simulink model "CMOS_Kernel_Memory_Sync"  (R2023b)
settings: Solver=VariableStepAuto  StartTime=0.0  StopTime=30000000  RelTol=1e-3
values from neighbouring files (symbols this model uses):
  AmountOfPixelsPerScanline = 400    [Kernel_Setup_Script.m]
  AmountOfRamBlocksScanlines = 5    [Kernel_Setup_Script.m]
  AmountOfRamBlocksScanlinesOffset = AmountOfRamBlocksScanlines - 1    (= 4)    [Kernel_Setup_Script.m]
  AmountOfScanlinePixels = 73700    [Kernel_Setup_Script.m]
  AmountOfScanlinePixelsOffset = AmountOfScanlinePixels - 1    (= 73699)    [Kernel_Setup_Script.m]
  AmountOfScanlines = 1100    [Kernel_Setup_Script.m]
  AmountOfScanlinesOffset = AmountOfScanlines - 1    (= 1099)    [Kernel_Setup_Script.m]
  AOPPK_Off = AmountOfPixelsPerScanline - 1    (= 399)    [Kernel_Setup_Script.m]
  AOPPS_Off = AmountOfPixelsPerScanline - 1    (= 399)    [Kernel_Setup_Script.m]
  FramePackOff_0 = FramePackOff_0 - ScanlineFifoCheck    [Kernel_Setup_Script.m]
  FramePackOff_1 = FramePackOff_1 - ScanlineFifoCheck    [Kernel_Setup_Script.m]
  FramePackOff_2 = FramePackOff_2 - ScanlineFifoCheck    [Kernel_Setup_Script.m]
  FramePackOff_3 = FramePackOff_3 - ScanlineFifoCheck    [Kernel_Setup_Script.m]
  FramePackOff_4 = FramePackOff_4 - ScanlineFifoCheck    [Kernel_Setup_Script.m]
  FramePackOff_5 = FramePackOff_5 - ScanlineFifoCheck    [Kernel_Setup_Script.m]
  KernelPackOff_0 = KernelPackOff_0 - KernelBitsPerRow    [Kernel_Setup_Script.m]
  KernelPackOff_1 = KernelPackOff_1 - KernelBitsPerRow    [Kernel_Setup_Script.m]
  KernelPackOff_2 = KernelPackOff_2 - KernelBitsPerRow    [Kernel_Setup_Script.m]
  KernelPackOff_3 = KernelPackOff_3 - KernelBitsPerRow    [Kernel_Setup_Script.m]
  Slice59DownTo48Top = (MsbOffset - (ScanlinePixelBitSizeController*1))    (= 59)    [Kernel_Setup_Script.m]
  Slice71DownTo60Top = (MsbOffset - (ScanlinePixelBitSizeController*0))    (= 71)    [Kernel_Setup_Script.m]
  TotalSectionsForFrames = AmountOfScanlines/AmountOfRamBlocksScanlines    (= 220)    [Kernel_Setup_Script.m]
  UltraRamRows = AmountOfPixelsPerScanline/ScanlineFifoCheck    [Kernel_Setup_Script.m]
  UltraRamRowsCeil = ceil(AmountOfPixelsPerScanline/ScanlineFifoCheck)    [Kernel_Setup_Script.m]
  UltraRamRowsKernel = AmountOfPixelsPerScanline/KernelBitsPerRow    (= 100)    [Kernel_Setup_Script.m]
  UltraRamRowsKernelCeil = ceil(AmountOfPixelsPerScanline/KernelBitsPerRow)    [Kernel_Setup_Script.m]
  UltraRamRowsMemorySectionOffset = UltraRamRowsCeil*AmountOfRamBlocksScanlines    [Kernel_Setup_Script.m]
  UltraRamRowsOffset = UltraRamRowsCeil - 1    [Kernel_Setup_Script.m]
undefined symbols (not defined in the file or in its folder): c, Down, sfvc784, Up, xck26
libraries: hdlBasic x4512, vmcUtilities x1
(part 38 of 39)

== system CMOS_Kernel_Memory_Sync/Memory Handler/Data Slicer/Kernel RAM Slicer/72 Bit Kernel Unpacker RAM 1/Unpack Kernel 72 Bit FIFO 0 ==
  72 Bit Input : Inport
  Slice 17 Down To 0 : hdlBasic/Slice  nbits=KernelWeightBitSizeController  boolean_output=off  mode=Upper Bit Location + Width  bit1=KernelSlice17DownTo0Top  base1=LSB of Input  bit0=0  base0=Binary Point of Input  XmcBlockStatus=1  maskContainerNames=group1  block_type=slice  block_config=sysgen:Slice_config
  Slice 35 Down To 18 : hdlBasic/Slice  nbits=KernelWeightBitSizeController  boolean_output=off  mode=Upper Bit Location + Width  bit1=KernelSlice35DownTo18Top  base1=LSB of Input  bit0=18  base0=Binary Point of Input  XmcBlockStatus=1  maskContainerNames=group1  block_type=slice  block_config=sysgen:Slice_config
  Slice 53 Down To 36 : hdlBasic/Slice  nbits=KernelWeightBitSizeController  boolean_output=off  mode=Upper Bit Location + Width  bit1=KernelSlice53DownTo36Top  base1=LSB of Input  bit0=36  base0=Binary Point of Input  XmcBlockStatus=1  maskContainerNames=group1  block_type=slice  block_config=sysgen:Slice_config
  Slice 71 Down To 54 : hdlBasic/Slice  nbits=KernelWeightBitSizeController  boolean_output=off  mode=Upper Bit Location + Width  bit1=KernelSlice71DownTo54Top  base1=LSB of Input  bit0=54  base0=Binary Point of Input  XmcBlockStatus=1  maskContainerNames=group1  block_type=slice  block_config=sysgen:Slice_config
  71 Downto 54 : Outport
  53 Downto 36 : Outport  Port=2
  35 Downto 18 : Outport  Port=3
  17 Downto 0 : Outport  Port=4
  wires:
  72 Bit Input/1 -> Slice 17 Down To 0/1, Slice 35 Down To 18/1, Slice 53 Down To 36/1, Slice 71 Down To 54/1
  Slice 35 Down To 18/1 -> 35 Downto 18/1
  Slice 53 Down To 36/1 -> 53 Downto 36/1
  Slice 17 Down To 0/1 -> 17 Downto 0/1
  Slice 71 Down To 54/1 -> 71 Downto 54/1

== system CMOS_Kernel_Memory_Sync/Memory Handler/Data Slicer/Kernel RAM Slicer/72 Bit Kernel Unpacker RAM 1/Unpack Kernel 72 Bit FIFO 1 ==
  72 Bit Input : Inport
  Slice 17 Down To 0 : hdlBasic/Slice  nbits=KernelWeightBitSizeController  boolean_output=off  mode=Upper Bit Location + Width  bit1=KernelSlice17DownTo0Top  base1=LSB of Input  bit0=0  base0=Binary Point of Input  XmcBlockStatus=1  maskContainerNames=group1  block_type=slice  block_config=sysgen:Slice_config
  Slice 35 Down To 18 : hdlBasic/Slice  nbits=KernelWeightBitSizeController  boolean_output=off  mode=Upper Bit Location + Width  bit1=KernelSlice35DownTo18Top  base1=LSB of Input  bit0=18  base0=Binary Point of Input  XmcBlockStatus=1  maskContainerNames=group1  block_type=slice  block_config=sysgen:Slice_config
  Slice 53 Down To 36 : hdlBasic/Slice  nbits=KernelWeightBitSizeController  boolean_output=off  mode=Upper Bit Location + Width  bit1=KernelSlice53DownTo36Top  base1=LSB of Input  bit0=36  base0=Binary Point of Input  XmcBlockStatus=1  maskContainerNames=group1  block_type=slice  block_config=sysgen:Slice_config
  Slice 71 Down To 54 : hdlBasic/Slice  nbits=KernelWeightBitSizeController  boolean_output=off  mode=Upper Bit Location + Width  bit1=KernelSlice71DownTo54Top  base1=LSB of Input  bit0=54  base0=Binary Point of Input  XmcBlockStatus=1  maskContainerNames=group1  block_type=slice  block_config=sysgen:Slice_config
  71 Downto 54 : Outport
  53 Downto 36 : Outport  Port=2
  35 Downto 18 : Outport  Port=3
  17 Downto 0 : Outport  Port=4
  wires:
  72 Bit Input/1 -> Slice 17 Down To 0/1, Slice 35 Down To 18/1, Slice 53 Down To 36/1, Slice 71 Down To 54/1
  Slice 35 Down To 18/1 -> 35 Downto 18/1
  Slice 53 Down To 36/1 -> 53 Downto 36/1
  Slice 17 Down To 0/1 -> 17 Downto 0/1
  Slice 71 Down To 54/1 -> 71 Downto 54/1

== system CMOS_Kernel_Memory_Sync/Memory Handler/Data Slicer/Kernel RAM Slicer/72 Bit Kernel Unpacker RAM 1/Unpack Kernel 72 Bit FIFO 2 ==
  72 Bit Input : Inport
  Slice 17 Down To 0 : hdlBasic/Slice  nbits=KernelWeightBitSizeController  boolean_output=off  mode=Upper Bit Location + Width  bit1=KernelSlice17DownTo0Top  base1=LSB of Input  bit0=0  base0=Binary Point of Input  XmcBlockStatus=1  maskContainerNames=group1  block_type=slice  block_config=sysgen:Slice_config
  Slice 35 Down To 18 : hdlBasic/Slice  nbits=KernelWeightBitSizeController  boolean_output=off  mode=Upper Bit Location + Width  bit1=KernelSlice35DownTo18Top  base1=LSB of Input  bit0=18  base0=Binary Point of Input  XmcBlockStatus=1  maskContainerNames=group1  block_type=slice  block_config=sysgen:Slice_config
  Slice 53 Down To 36 : hdlBasic/Slice  nbits=KernelWeightBitSizeController  boolean_output=off  mode=Upper Bit Location + Width  bit1=KernelSlice53DownTo36Top  base1=LSB of Input  bit0=36  base0=Binary Point of Input  XmcBlockStatus=1  maskContainerNames=group1  block_type=slice  block_config=sysgen:Slice_config
  Slice 71 Down To 54 : hdlBasic/Slice  nbits=KernelWeightBitSizeController  boolean_output=off  mode=Upper Bit Location + Width  bit1=KernelSlice71DownTo54Top  base1=LSB of Input  bit0=54  base0=Binary Point of Input  XmcBlockStatus=1  maskContainerNames=group1  block_type=slice  block_config=sysgen:Slice_config
  71 Downto 54 : Outport
  53 Downto 36 : Outport  Port=2
  35 Downto 18 : Outport  Port=3
  17 Downto 0 : Outport  Port=4
  wires:
  72 Bit Input/1 -> Slice 17 Down To 0/1, Slice 35 Down To 18/1, Slice 53 Down To 36/1, Slice 71 Down To 54/1
  Slice 35 Down To 18/1 -> 35 Downto 18/1
  Slice 53 Down To 36/1 -> 53 Downto 36/1
  Slice 17 Down To 0/1 -> 17 Downto 0/1
  Slice 71 Down To 54/1 -> 71 Downto 54/1

== system CMOS_Kernel_Memory_Sync/Memory Handler/Data Slicer/Kernel RAM Slicer/72 Bit Kernel Unpacker RAM 2/Unpack Kernel 72 Bit FIFO 0 ==
  72 Bit Input : Inport
  Slice 17 Down To 0 : hdlBasic/Slice  nbits=KernelWeightBitSizeController  boolean_output=off  mode=Upper Bit Location + Width  bit1=KernelSlice17DownTo0Top  base1=LSB of Input  bit0=0  base0=Binary Point of Input  XmcBlockStatus=1  maskContainerNames=group1  block_type=slice  block_config=sysgen:Slice_config
  Slice 35 Down To 18 : hdlBasic/Slice  nbits=KernelWeightBitSizeController  boolean_output=off  mode=Upper Bit Location + Width  bit1=KernelSlice35DownTo18Top  base1=LSB of Input  bit0=18  base0=Binary Point of Input  XmcBlockStatus=1  maskContainerNames=group1  block_type=slice  block_config=sysgen:Slice_config
  Slice 53 Down To 36 : hdlBasic/Slice  nbits=KernelWeightBitSizeController  boolean_output=off  mode=Upper Bit Location + Width  bit1=KernelSlice53DownTo36Top  base1=LSB of Input  bit0=36  base0=Binary Point of Input  XmcBlockStatus=1  maskContainerNames=group1  block_type=slice  block_config=sysgen:Slice_config
  Slice 71 Down To 54 : hdlBasic/Slice  nbits=KernelWeightBitSizeController  boolean_output=off  mode=Upper Bit Location + Width  bit1=KernelSlice71DownTo54Top  base1=LSB of Input  bit0=54  base0=Binary Point of Input  XmcBlockStatus=1  maskContainerNames=group1  block_type=slice  block_config=sysgen:Slice_config
  71 Downto 54 : Outport
  53 Downto 36 : Outport  Port=2
  35 Downto 18 : Outport  Port=3
  17 Downto 0 : Outport  Port=4
  wires:
  72 Bit Input/1 -> Slice 17 Down To 0/1, Slice 35 Down To 18/1, Slice 53 Down To 36/1, Slice 71 Down To 54/1
  Slice 35 Down To 18/1 -> 35 Downto 18/1
  Slice 53 Down To 36/1 -> 53 Downto 36/1
  Slice 17 Down To 0/1 -> 17 Downto 0/1
  Slice 71 Down To 54/1 -> 71 Downto 54/1

== system CMOS_Kernel_Memory_Sync/Memory Handler/Data Slicer/Kernel RAM Slicer/72 Bit Kernel Unpacker RAM 2/Unpack Kernel 72 Bit FIFO 1 ==
  72 Bit Input : Inport
  Slice 17 Down To 0 : hdlBasic/Slice  nbits=KernelWeightBitSizeController  boolean_output=off  mode=Upper Bit Location + Width  bit1=KernelSlice17DownTo0Top  base1=LSB of Input  bit0=0  base0=Binary Point of Input  XmcBlockStatus=1  maskContainerNames=group1  block_type=slice  block_config=sysgen:Slice_config
  Slice 35 Down To 18 : hdlBasic/Slice  nbits=KernelWeightBitSizeController  boolean_output=off  mode=Upper Bit Location + Width  bit1=KernelSlice35DownTo18Top  base1=LSB of Input  bit0=18  base0=Binary Point of Input  XmcBlockStatus=1  maskContainerNames=group1  block_type=slice  block_config=sysgen:Slice_config
  Slice 53 Down To 36 : hdlBasic/Slice  nbits=KernelWeightBitSizeController  boolean_output=off  mode=Upper Bit Location + Width  bit1=KernelSlice53DownTo36Top  base1=LSB of Input  bit0=36  base0=Binary Point of Input  XmcBlockStatus=1  maskContainerNames=group1  block_type=slice  block_config=sysgen:Slice_config
  Slice 71 Down To 54 : hdlBasic/Slice  nbits=KernelWeightBitSizeController  boolean_output=off  mode=Upper Bit Location + Width  bit1=KernelSlice71DownTo54Top  base1=LSB of Input  bit0=54  base0=Binary Point of Input  XmcBlockStatus=1  maskContainerNames=group1  block_type=slice  block_config=sysgen:Slice_config
  71 Downto 54 : Outport
  53 Downto 36 : Outport  Port=2
  35 Downto 18 : Outport  Port=3
  17 Downto 0 : Outport  Port=4
  wires:
  72 Bit Input/1 -> Slice 17 Down To 0/1, Slice 35 Down To 18/1, Slice 53 Down To 36/1, Slice 71 Down To 54/1
  Slice 35 Down To 18/1 -> 35 Downto 18/1
  Slice 53 Down To 36/1 -> 53 Downto 36/1
  Slice 17 Down To 0/1 -> 17 Downto 0/1
  Slice 71 Down To 54/1 -> 71 Downto 54/1

== system CMOS_Kernel_Memory_Sync/Memory Handler/Data Slicer/Kernel RAM Slicer/72 Bit Kernel Unpacker RAM 2/Unpack Kernel 72 Bit FIFO 2 ==
  72 Bit Input : Inport
  Slice 17 Down To 0 : hdlBasic/Slice  nbits=KernelWeightBitSizeController  boolean_output=off  mode=Upper Bit Location + Width  bit1=KernelSlice17DownTo0Top  base1=LSB of Input  bit0=0  base0=Binary Point of Input  XmcBlockStatus=1  maskContainerNames=group1  block_type=slice  block_config=sysgen:Slice_config
  Slice 35 Down To 18 : hdlBasic/Slice  nbits=KernelWeightBitSizeController  boolean_output=off  mode=Upper Bit Location + Width  bit1=KernelSlice35DownTo18Top  base1=LSB of Input  bit0=18  base0=Binary Point of Input  XmcBlockStatus=1  maskContainerNames=group1  block_type=slice  block_config=sysgen:Slice_config
  Slice 53 Down To 36 : hdlBasic/Slice  nbits=KernelWeightBitSizeController  boolean_output=off  mode=Upper Bit Location + Width  bit1=KernelSlice53DownTo36Top  base1=LSB of Input  bit0=36  base0=Binary Point of Input  XmcBlockStatus=1  maskContainerNames=group1  block_type=slice  block_config=sysgen:Slice_config
  Slice 71 Down To 54 : hdlBasic/Slice  nbits=KernelWeightBitSizeController  boolean_output=off  mode=Upper Bit Location + Width  bit1=KernelSlice71DownTo54Top  base1=LSB of Input  bit0=54  base0=Binary Point of Input  XmcBlockStatus=1  maskContainerNames=group1  block_type=slice  block_config=sysgen:Slice_config
  71 Downto 54 : Outport
  53 Downto 36 : Outport  Port=2
  35 Downto 18 : Outport  Port=3
  17 Downto 0 : Outport  Port=4
  wires:
  72 Bit Input/1 -> Slice 17 Down To 0/1, Slice 35 Down To 18/1, Slice 53 Down To 36/1, Slice 71 Down To 54/1
  Slice 35 Down To 18/1 -> 35 Downto 18/1
  Slice 53 Down To 36/1 -> 53 Downto 36/1
  Slice 17 Down To 0/1 -> 17 Downto 0/1
  Slice 71 Down To 54/1 -> 71 Downto 54/1

== system CMOS_Kernel_Memory_Sync/Memory Handler/Data Slicer/Kernel RAM Slicer/72 Bit Kernel Unpacker RAM 3/Unpack Kernel 72 Bit FIFO 0 ==
  72 Bit Input : Inport
  Slice 17 Down To 0 : hdlBasic/Slice  nbits=KernelWeightBitSizeController  boolean_output=off  mode=Upper Bit Location + Width  bit1=KernelSlice17DownTo0Top  base1=LSB of Input  bit0=0  base0=Binary Point of Input  XmcBlockStatus=1  maskContainerNames=group1  block_type=slice  block_config=sysgen:Slice_config
  Slice 35 Down To 18 : hdlBasic/Slice  nbits=KernelWeightBitSizeController  boolean_output=off  mode=Upper Bit Location + Width  bit1=KernelSlice35DownTo18Top  base1=LSB of Input  bit0=18  base0=Binary Point of Input  XmcBlockStatus=1  maskContainerNames=group1  block_type=slice  block_config=sysgen:Slice_config
  Slice 53 Down To 36 : hdlBasic/Slice  nbits=KernelWeightBitSizeController  boolean_output=off  mode=Upper Bit Location + Width  bit1=KernelSlice53DownTo36Top  base1=LSB of Input  bit0=36  base0=Binary Point of Input  XmcBlockStatus=1  maskContainerNames=group1  block_type=slice  block_config=sysgen:Slice_config
  Slice 71 Down To 54 : hdlBasic/Slice  nbits=KernelWeightBitSizeController  boolean_output=off  mode=Upper Bit Location + Width  bit1=KernelSlice71DownTo54Top  base1=LSB of Input  bit0=54  base0=Binary Point of Input  XmcBlockStatus=1  maskContainerNames=group1  block_type=slice  block_config=sysgen:Slice_config
  71 Downto 54 : Outport
  53 Downto 36 : Outport  Port=2
  35 Downto 18 : Outport  Port=3
  17 Downto 0 : Outport  Port=4
  wires:
  72 Bit Input/1 -> Slice 17 Down To 0/1, Slice 35 Down To 18/1, Slice 53 Down To 36/1, Slice 71 Down To 54/1
  Slice 35 Down To 18/1 -> 35 Downto 18/1
  Slice 53 Down To 36/1 -> 53 Downto 36/1
  Slice 17 Down To 0/1 -> 17 Downto 0/1
  Slice 71 Down To 54/1 -> 71 Downto 54/1

== system CMOS_Kernel_Memory_Sync/Memory Handler/Data Slicer/Kernel RAM Slicer/72 Bit Kernel Unpacker RAM 3/Unpack Kernel 72 Bit FIFO 1 ==
  72 Bit Input : Inport
  Slice 17 Down To 0 : hdlBasic/Slice  nbits=KernelWeightBitSizeController  boolean_output=off  mode=Upper Bit Location + Width  bit1=KernelSlice17DownTo0Top  base1=LSB of Input  bit0=0  base0=Binary Point of Input  XmcBlockStatus=1  maskContainerNames=group1  block_type=slice  block_config=sysgen:Slice_config
  Slice 35 Down To 18 : hdlBasic/Slice  nbits=KernelWeightBitSizeController  boolean_output=off  mode=Upper Bit Location + Width  bit1=KernelSlice35DownTo18Top  base1=LSB of Input  bit0=18  base0=Binary Point of Input  XmcBlockStatus=1  maskContainerNames=group1  block_type=slice  block_config=sysgen:Slice_config
  Slice 53 Down To 36 : hdlBasic/Slice  nbits=KernelWeightBitSizeController  boolean_output=off  mode=Upper Bit Location + Width  bit1=KernelSlice53DownTo36Top  base1=LSB of Input  bit0=36  base0=Binary Point of Input  XmcBlockStatus=1  maskContainerNames=group1  block_type=slice  block_config=sysgen:Slice_config
  Slice 71 Down To 54 : hdlBasic/Slice  nbits=KernelWeightBitSizeController  boolean_output=off  mode=Upper Bit Location + Width  bit1=KernelSlice71DownTo54Top  base1=LSB of Input  bit0=54  base0=Binary Point of Input  XmcBlockStatus=1  maskContainerNames=group1  block_type=slice  block_config=sysgen:Slice_config
  71 Downto 54 : Outport
  53 Downto 36 : Outport  Port=2
  35 Downto 18 : Outport  Port=3
  17 Downto 0 : Outport  Port=4
  wires:
  72 Bit Input/1 -> Slice 17 Down To 0/1, Slice 35 Down To 18/1, Slice 53 Down To 36/1, Slice 71 Down To 54/1
  Slice 35 Down To 18/1 -> 35 Downto 18/1
  Slice 53 Down To 36/1 -> 53 Downto 36/1
  Slice 17 Down To 0/1 -> 17 Downto 0/1
  Slice 71 Down To 54/1 -> 71 Downto 54/1

== system CMOS_Kernel_Memory_Sync/Memory Handler/Data Slicer/Kernel RAM Slicer/72 Bit Kernel Unpacker RAM 3/Unpack Kernel 72 Bit FIFO 2 ==
  72 Bit Input : Inport
  Slice 17 Down To 0 : hdlBasic/Slice  nbits=KernelWeightBitSizeController  boolean_output=off  mode=Upper Bit Location + Width  bit1=KernelSlice17DownTo0Top  base1=LSB of Input  bit0=0  base0=Binary Point of Input  XmcBlockStatus=1  maskContainerNames=group1  block_type=slice  block_config=sysgen:Slice_config
  Slice 35 Down To 18 : hdlBasic/Slice  nbits=KernelWeightBitSizeController  boolean_output=off  mode=Upper Bit Location + Width  bit1=KernelSlice35DownTo18Top  base1=LSB of Input  bit0=18  base0=Binary Point of Input  XmcBlockStatus=1  maskContainerNames=group1  block_type=slice  block_config=sysgen:Slice_config
  Slice 53 Down To 36 : hdlBasic/Slice  nbits=KernelWeightBitSizeController  boolean_output=off  mode=Upper Bit Location + Width  bit1=KernelSlice53DownTo36Top  base1=LSB of Input  bit0=36  base0=Binary Point of Input  XmcBlockStatus=1  maskContainerNames=group1  block_type=slice  block_config=sysgen:Slice_config
  Slice 71 Down To 54 : hdlBasic/Slice  nbits=KernelWeightBitSizeController  boolean_output=off  mode=Upper Bit Location + Width  bit1=KernelSlice71DownTo54Top  base1=LSB of Input  bit0=54  base0=Binary Point of Input  XmcBlockStatus=1  maskContainerNames=group1  block_type=slice  block_config=sysgen:Slice_config
  71 Downto 54 : Outport
  53 Downto 36 : Outport  Port=2
  35 Downto 18 : Outport  Port=3
  17 Downto 0 : Outport  Port=4
  wires:
  72 Bit Input/1 -> Slice 17 Down To 0/1, Slice 35 Down To 18/1, Slice 53 Down To 36/1, Slice 71 Down To 54/1
  Slice 35 Down To 18/1 -> 35 Downto 18/1
  Slice 53 Down To 36/1 -> 53 Downto 36/1
  Slice 17 Down To 0/1 -> 17 Downto 0/1
  Slice 71 Down To 54/1 -> 71 Downto 54/1

== system CMOS_Kernel_Memory_Sync/Memory Handler/Data Slicer/Kernel RAM Slicer/72 Bit Kernel Unpacker RAM 4/Unpack Kernel 72 Bit FIFO 0 ==
  72 Bit Input : Inport
  Slice 17 Down To 0 : hdlBasic/Slice  nbits=KernelWeightBitSizeController  boolean_output=off  mode=Upper Bit Location + Width  bit1=KernelSlice17DownTo0Top  base1=LSB of Input  bit0=0  base0=Binary Point of Input  XmcBlockStatus=1  maskContainerNames=group1  block_type=slice  block_config=sysgen:Slice_config
  Slice 35 Down To 18 : hdlBasic/Slice  nbits=KernelWeightBitSizeController  boolean_output=off  mode=Upper Bit Location + Width  bit1=KernelSlice35DownTo18Top  base1=LSB of Input  bit0=18  base0=Binary Point of Input  XmcBlockStatus=1  maskContainerNames=group1  block_type=slice  block_config=sysgen:Slice_config
  Slice 53 Down To 36 : hdlBasic/Slice  nbits=KernelWeightBitSizeController  boolean_output=off  mode=Upper Bit Location + Width  bit1=KernelSlice53DownTo36Top  base1=LSB of Input  bit0=36  base0=Binary Point of Input  XmcBlockStatus=1  maskContainerNames=group1  block_type=slice  block_config=sysgen:Slice_config
  Slice 71 Down To 54 : hdlBasic/Slice  nbits=KernelWeightBitSizeController  boolean_output=off  mode=Upper Bit Location + Width  bit1=KernelSlice71DownTo54Top  base1=LSB of Input  bit0=54  base0=Binary Point of Input  XmcBlockStatus=1  maskContainerNames=group1  block_type=slice  block_config=sysgen:Slice_config
  71 Downto 54 : Outport
  53 Downto 36 : Outport  Port=2
  35 Downto 18 : Outport  Port=3
  17 Downto 0 : Outport  Port=4
  wires:
  72 Bit Input/1 -> Slice 17 Down To 0/1, Slice 35 Down To 18/1, Slice 53 Down To 36/1, Slice 71 Down To 54/1
  Slice 35 Down To 18/1 -> 35 Downto 18/1
  Slice 53 Down To 36/1 -> 53 Downto 36/1
  Slice 17 Down To 0/1 -> 17 Downto 0/1
  Slice 71 Down To 54/1 -> 71 Downto 54/1

== system CMOS_Kernel_Memory_Sync/Memory Handler/Data Slicer/Kernel RAM Slicer/72 Bit Kernel Unpacker RAM 4/Unpack Kernel 72 Bit FIFO 1 ==
  72 Bit Input : Inport
  Slice 17 Down To 0 : hdlBasic/Slice  nbits=KernelWeightBitSizeController  boolean_output=off  mode=Upper Bit Location + Width  bit1=KernelSlice17DownTo0Top  base1=LSB of Input  bit0=0  base0=Binary Point of Input  XmcBlockStatus=1  maskContainerNames=group1  block_type=slice  block_config=sysgen:Slice_config
  Slice 35 Down To 18 : hdlBasic/Slice  nbits=KernelWeightBitSizeController  boolean_output=off  mode=Upper Bit Location + Width  bit1=KernelSlice35DownTo18Top  base1=LSB of Input  bit0=18  base0=Binary Point of Input  XmcBlockStatus=1  maskContainerNames=group1  block_type=slice  block_config=sysgen:Slice_config
  Slice 53 Down To 36 : hdlBasic/Slice  nbits=KernelWeightBitSizeController  boolean_output=off  mode=Upper Bit Location + Width  bit1=KernelSlice53DownTo36Top  base1=LSB of Input  bit0=36  base0=Binary Point of Input  XmcBlockStatus=1  maskContainerNames=group1  block_type=slice  block_config=sysgen:Slice_config
  Slice 71 Down To 54 : hdlBasic/Slice  nbits=KernelWeightBitSizeController  boolean_output=off  mode=Upper Bit Location + Width  bit1=KernelSlice71DownTo54Top  base1=LSB of Input  bit0=54  base0=Binary Point of Input  XmcBlockStatus=1  maskContainerNames=group1  block_type=slice  block_config=sysgen:Slice_config
  71 Downto 54 : Outport
  53 Downto 36 : Outport  Port=2
  35 Downto 18 : Outport  Port=3
  17 Downto 0 : Outport  Port=4
  wires:
  72 Bit Input/1 -> Slice 17 Down To 0/1, Slice 35 Down To 18/1, Slice 53 Down To 36/1, Slice 71 Down To 54/1
  Slice 35 Down To 18/1 -> 35 Downto 18/1
  Slice 53 Down To 36/1 -> 53 Downto 36/1
  Slice 17 Down To 0/1 -> 17 Downto 0/1
  Slice 71 Down To 54/1 -> 71 Downto 54/1

== system CMOS_Kernel_Memory_Sync/Memory Handler/Data Slicer/Kernel RAM Slicer/72 Bit Kernel Unpacker RAM 4/Unpack Kernel 72 Bit FIFO 2 ==
  72 Bit Input : Inport
  Slice 17 Down To 0 : hdlBasic/Slice  nbits=KernelWeightBitSizeController  boolean_output=off  mode=Upper Bit Location + Width  bit1=KernelSlice17DownTo0Top  base1=LSB of Input  bit0=0  base0=Binary Point of Input  XmcBlockStatus=1  maskContainerNames=group1  block_type=slice  block_config=sysgen:Slice_config
  Slice 35 Down To 18 : hdlBasic/Slice  nbits=KernelWeightBitSizeController  boolean_output=off  mode=Upper Bit Location + Width  bit1=KernelSlice35DownTo18Top  base1=LSB of Input  bit0=18  base0=Binary Point of Input  XmcBlockStatus=1  maskContainerNames=group1  block_type=slice  block_config=sysgen:Slice_config
  Slice 53 Down To 36 : hdlBasic/Slice  nbits=KernelWeightBitSizeController  boolean_output=off  mode=Upper Bit Location + Width  bit1=KernelSlice53DownTo36Top  base1=LSB of Input  bit0=36  base0=Binary Point of Input  XmcBlockStatus=1  maskContainerNames=group1  block_type=slice  block_config=sysgen:Slice_config
  Slice 71 Down To 54 : hdlBasic/Slice  nbits=KernelWeightBitSizeController  boolean_output=off  mode=Upper Bit Location + Width  bit1=KernelSlice71DownTo54Top  base1=LSB of Input  bit0=54  base0=Binary Point of Input  XmcBlockStatus=1  maskContainerNames=group1  block_type=slice  block_config=sysgen:Slice_config
  71 Downto 54 : Outport
  53 Downto 36 : Outport  Port=2
  35 Downto 18 : Outport  Port=3
  17 Downto 0 : Outport  Port=4
  wires:
  72 Bit Input/1 -> Slice 17 Down To 0/1, Slice 35 Down To 18/1, Slice 53 Down To 36/1, Slice 71 Down To 54/1
  Slice 35 Down To 18/1 -> 35 Downto 18/1
  Slice 53 Down To 36/1 -> 53 Downto 36/1
  Slice 17 Down To 0/1 -> 17 Downto 0/1
  Slice 71 Down To 54/1 -> 71 Downto 54/1

== system CMOS_Kernel_Memory_Sync/Memory Handler/Math/Kernel Organizer/Determine Calculations Delay 1/Result Muxer 0 ==
  Select : Inport
  Valid : Inport  Port=2
  Force Off : Inport  Port=3
  Case 0 : hdlBasic/Mux  inputs=2  en=off  latency=1  precision=Full  arith_type=Unsigned  n_bits=16  bin_pt=14  quantization=Truncate  overflow=Wrap  XmcBlockStatus=1  maskContainerNames=tabcontainer1  block_type=mux  block_config=sysgen:Mux_config
  Case 1 : hdlBasic/Mux  inputs=2  en=off  latency=1  precision=Full  arith_type=Unsigned  n_bits=16  bin_pt=14  quantization=Truncate  overflow=Wrap  XmcBlockStatus=1  maskContainerNames=tabcontainer1  block_type=mux  block_config=sysgen:Mux_config
  Delay Valid 0 : hdlBasic/Delay  rst=off  en=off  latency=1  reg_retiming=off  XmcBlockStatus=1  maskContainerNames=group1  block_type=delay  block_config=sysgen:Delay_config
  Enable Passthrough Case 0 : hdlBasic/Logical  logical_function=AND  inputs=3  en=off  latency=1  precision=Full  arith_type=Unsigned  n_bits=16  bin_pt=0  align_bp=on  overflow=[]  quantization=[]  XmcBlockStatus=1  maskContainerNames=tabcontainer1  block_type=logical  block_config=sysgen:Logical_config
  Enable Passthrough Case 1 : hdlBasic/Logical  logical_function=AND  inputs=3  en=off  latency=1  precision=Full  arith_type=Unsigned  n_bits=16  bin_pt=0  align_bp=on  overflow=[]  quantization=[]  XmcBlockStatus=1  maskContainerNames=tabcontainer1  block_type=logical  block_config=sysgen:Logical_config
  Force Off MUX : hdlBasic/Mux  inputs=2  en=off  latency=1  precision=Full  arith_type=Unsigned  n_bits=16  bin_pt=14  quantization=Truncate  overflow=Wrap  XmcBlockStatus=1  maskContainerNames=tabcontainer1  block_type=mux  block_config=sysgen:Mux_config
  Off : hdlBasic/Constant  const=0  gui_display_data_type=Boolean  arith_type=Boolean  n_bits=16  bin_pt=14  preci_type=Single  exp_width=8  frac_width=24  explicit_period=off  period=1  XmcBlockStatus=1  maskContainerNames=tabcontainer1  block_type=constant  block_config=sysgen:Constant_config
  On : hdlBasic/Constant  const=1.0  gui_display_data_type=Boolean  arith_type=Boolean  n_bits=16  bin_pt=14  preci_type=Single  exp_width=8  frac_width=24  explicit_period=off  period=1  XmcBlockStatus=1  maskContainerNames=tabcontainer1  block_type=constant  block_config=sysgen:Constant_config
  Kernel Result Slice 0 Valid : Outport
  Kernel Result Slice 1 Valid : Outport  Port=2
  Kernel Result Slice 2 Valid : Outport  Port=3
  Kernel Result Slice 3 Valid : Outport  Port=4
  Kernel Result Slice 4 Valid : Outport  Port=5
  wires:
  Select/1 -> Case 0/1, Case 1/1
  Force Off/1 -> Force Off MUX/1
  On/1 -> Case 0/2, Force Off MUX/2, Case 1/3
  Off/1 -> Force Off MUX/3, Case 1/2, Case 0/3
  Valid/1 -> Delay Valid 0/1
  Case 0/1 -> Enable Passthrough Case 0/1
  Case 1/1 -> Enable Passthrough Case 1/1
  Delay Valid 0/1 -> Enable Passthrough Case 1/2, Enable Passthrough Case 0/2
  Force Off MUX/1 -> Enable Passthrough Case 0/3, Enable Passthrough Case 1/3
  Enable Passthrough Case 0/1 -> Kernel Result Slice 3 Valid/1, Kernel Result Slice 4 Valid/1, Kernel Result Slice 2 Valid/1, Kernel Result Slice 1 Valid/1, Kernel Result Slice 0 Valid/1

== system CMOS_Kernel_Memory_Sync/Memory Handler/Math/Kernel Organizer/Determine Calculations Delay 1/Result Muxer 1 ==
  Select : Inport
  Valid : Inport  Port=2
  Case 0 : hdlBasic/Mux  inputs=2  en=off  latency=1  precision=Full  arith_type=Unsigned  n_bits=16  bin_pt=14  quantization=Truncate  overflow=Wrap  XmcBlockStatus=1  maskContainerNames=tabcontainer1  block_type=mux  block_config=sysgen:Mux_config
  Case 1 : hdlBasic/Mux  inputs=2  en=off  latency=1  precision=Full  arith_type=Unsigned  n_bits=16  bin_pt=14  quantization=Truncate  overflow=Wrap  XmcBlockStatus=1  maskContainerNames=tabcontainer1  block_type=mux  block_config=sysgen:Mux_config
  Delay Valid 0 : hdlBasic/Delay  rst=off  en=off  latency=1  reg_retiming=off  XmcBlockStatus=1  maskContainerNames=group1  block_type=delay  block_config=sysgen:Delay_config
  Enable Passthrough Case 0 : hdlBasic/Logical  logical_function=AND  inputs=2  en=off  latency=1  precision=Full  arith_type=Unsigned  n_bits=16  bin_pt=0  align_bp=on  overflow=[]  quantization=[]  XmcBlockStatus=1  maskContainerNames=tabcontainer1  block_type=logical  block_config=sysgen:Logical_config
  Enable Passthrough Case 1 : hdlBasic/Logical  logical_function=AND  inputs=2  en=off  latency=1  precision=Full  arith_type=Unsigned  n_bits=16  bin_pt=0  align_bp=on  overflow=[]  quantization=[]  XmcBlockStatus=1  maskContainerNames=tabcontainer1  block_type=logical  block_config=sysgen:Logical_config
  Off : hdlBasic/Constant  const=0  gui_display_data_type=Boolean  arith_type=Boolean  n_bits=16  bin_pt=14  preci_type=Single  exp_width=8  frac_width=24  explicit_period=off  period=1  XmcBlockStatus=1  maskContainerNames=tabcontainer1  block_type=constant  block_config=sysgen:Constant_config
  On : hdlBasic/Constant  const=1.0  gui_display_data_type=Boolean  arith_type=Boolean  n_bits=16  bin_pt=14  preci_type=Single  exp_width=8  frac_width=24  explicit_period=off  period=1  XmcBlockStatus=1  maskContainerNames=tabcontainer1  block_type=constant  block_config=sysgen:Constant_config
  Kernel Result Slice 0 Valid : Outport
  Kernel Result Slice 1 Valid : Outport  Port=2
  Kernel Result Slice 2 Valid : Outport  Port=3
  Kernel Result Slice 3 Valid : Outport  Port=4
  Kernel Result Slice 4 Valid : Outport  Port=5
  wires:
  Select/1 -> Case 0/1, Case 1/1
  On/1 -> Case 0/2, Case 1/3
  Off/1 -> Case 1/2, Case 0/3
  Valid/1 -> Delay Valid 0/1
  Case 0/1 -> Enable Passthrough Case 0/1
  Case 1/1 -> Enable Passthrough Case 1/1
  Delay Valid 0/1 -> Enable Passthrough Case 1/2, Enable Passthrough Case 0/2
  Enable Passthrough Case 0/1 -> Kernel Result Slice 3 Valid/1, Kernel Result Slice 2 Valid/1, Kernel Result Slice 1 Valid/1, Kernel Result Slice 0 Valid/1
  Enable Passthrough Case 1/1 -> Kernel Result Slice 4 Valid/1

== system CMOS_Kernel_Memory_Sync/Memory Handler/Math/Kernel Organizer/Determine Calculations Delay 1/Result Muxer 2 ==
  Select : Inport
  Valid : Inport  Port=2
  Case 0 : hdlBasic/Mux  inputs=2  en=off  latency=1  precision=Full  arith_type=Unsigned  n_bits=16  bin_pt=14  quantization=Truncate  overflow=Wrap  XmcBlockStatus=1  maskContainerNames=tabcontainer1  block_type=mux  block_config=sysgen:Mux_config
  Case 1 : hdlBasic/Mux  inputs=2  en=off  latency=1  precision=Full  arith_type=Unsigned  n_bits=16  bin_pt=14  quantization=Truncate  overflow=Wrap  XmcBlockStatus=1  maskContainerNames=tabcontainer1  block_type=mux  block_config=sysgen:Mux_config
  Delay Valid 0 : hdlBasic/Delay  rst=off  en=off  latency=1  reg_retiming=off  XmcBlockStatus=1  maskContainerNames=group1  block_type=delay  block_config=sysgen:Delay_config
  Enable Passthrough Case 0 : hdlBasic/Logical  logical_function=AND  inputs=2  en=off  latency=1  precision=Full  arith_type=Unsigned  n_bits=16  bin_pt=0  align_bp=on  overflow=[]  quantization=[]  XmcBlockStatus=1  maskContainerNames=tabcontainer1  block_type=logical  block_config=sysgen:Logical_config
  Enable Passthrough Case 1 : hdlBasic/Logical  logical_function=AND  inputs=2  en=off  latency=1  precision=Full  arith_type=Unsigned  n_bits=16  bin_pt=0  align_bp=on  overflow=[]  quantization=[]  XmcBlockStatus=1  maskContainerNames=tabcontainer1  block_type=logical  block_config=sysgen:Logical_config
  Off : hdlBasic/Constant  const=0  gui_display_data_type=Boolean  arith_type=Boolean  n_bits=16  bin_pt=14  preci_type=Single  exp_width=8  frac_width=24  explicit_period=off  period=1  XmcBlockStatus=1  maskContainerNames=tabcontainer1  block_type=constant  block_config=sysgen:Constant_config
  On : hdlBasic/Constant  const=1.0  gui_display_data_type=Boolean  arith_type=Boolean  n_bits=16  bin_pt=14  preci_type=Single  exp_width=8  frac_width=24  explicit_period=off  period=1  XmcBlockStatus=1  maskContainerNames=tabcontainer1  block_type=constant  block_config=sysgen:Constant_config
  Kernel Result Slice 0 Valid : Outport
  Kernel Result Slice 1 Valid : Outport  Port=2
  Kernel Result Slice 2 Valid : Outport  Port=3
  Kernel Result Slice 3 Valid : Outport  Port=4
  Kernel Result Slice 4 Valid : Outport  Port=5
  wires:
  Select/1 -> Case 0/1, Case 1/1
  On/1 -> Case 0/2, Case 1/3
  Off/1 -> Case 1/2, Case 0/3
  Valid/1 -> Delay Valid 0/1
  Case 0/1 -> Enable Passthrough Case 0/1
  Case 1/1 -> Enable Passthrough Case 1/1
  Delay Valid 0/1 -> Enable Passthrough Case 1/2, Enable Passthrough Case 0/2
  Enable Passthrough Case 0/1 -> Kernel Result Slice 2 Valid/1, Kernel Result Slice 1 Valid/1, Kernel Result Slice 0 Valid/1
  Enable Passthrough Case 1/1 -> Kernel Result Slice 3 Valid/1, Kernel Result Slice 4 Valid/1

== system CMOS_Kernel_Memory_Sync/Memory Handler/Math/Kernel Organizer/Determine Calculations Delay 1/Result Muxer 3 ==
  Select : Inport
  Valid : Inport  Port=2
  Case 0 : hdlBasic/Mux  inputs=2  en=off  latency=1  precision=Full  arith_type=Unsigned  n_bits=16  bin_pt=14  quantization=Truncate  overflow=Wrap  XmcBlockStatus=1  maskContainerNames=tabcontainer1  block_type=mux  block_config=sysgen:Mux_config
  Case 1 : hdlBasic/Mux  inputs=2  en=off  latency=1  precision=Full  arith_type=Unsigned  n_bits=16  bin_pt=14  quantization=Truncate  overflow=Wrap  XmcBlockStatus=1  maskContainerNames=tabcontainer1  block_type=mux  block_config=sysgen:Mux_config
  Delay Valid 0 : hdlBasic/Delay  rst=off  en=off  latency=1  reg_retiming=off  XmcBlockStatus=1  maskContainerNames=group1  block_type=delay  block_config=sysgen:Delay_config
  Enable Passthrough Case 0 : hdlBasic/Logical  logical_function=AND  inputs=2  en=off  latency=1  precision=Full  arith_type=Unsigned  n_bits=16  bin_pt=0  align_bp=on  overflow=[]  quantization=[]  XmcBlockStatus=1  maskContainerNames=tabcontainer1  block_type=logical  block_config=sysgen:Logical_config
  Enable Passthrough Case 1 : hdlBasic/Logical  logical_function=AND  inputs=2  en=off  latency=1  precision=Full  arith_type=Unsigned  n_bits=16  bin_pt=0  align_bp=on  overflow=[]  quantization=[]  XmcBlockStatus=1  maskContainerNames=tabcontainer1  block_type=logical  block_config=sysgen:Logical_config
  Off : hdlBasic/Constant  const=0  gui_display_data_type=Boolean  arith_type=Boolean  n_bits=16  bin_pt=14  preci_type=Single  exp_width=8  frac_width=24  explicit_period=off  period=1  XmcBlockStatus=1  maskContainerNames=tabcontainer1  block_type=constant  block_config=sysgen:Constant_config
  On : hdlBasic/Constant  const=1.0  gui_display_data_type=Boolean  arith_type=Boolean  n_bits=16  bin_pt=14  preci_type=Single  exp_width=8  frac_width=24  explicit_period=off  period=1  XmcBlockStatus=1  maskContainerNames=tabcontainer1  block_type=constant  block_config=sysgen:Constant_config
  Kernel Result Slice 0 Valid : Outport
  Kernel Result Slice 1 Valid : Outport  Port=2
  Kernel Result Slice 2 Valid : Outport  Port=3
  Kernel Result Slice 3 Valid : Outport  Port=4
  Kernel Result Slice 4 Valid : Outport  Port=5
  wires:
  Select/1 -> Case 0/1, Case 1/1
  On/1 -> Case 0/2, Case 1/3
  Off/1 -> Case 1/2, Case 0/3
  Valid/1 -> Delay Valid 0/1
  Case 0/1 -> Enable Passthrough Case 0/1
  Case 1/1 -> Enable Passthrough Case 1/1
  Delay Valid 0/1 -> Enable Passthrough Case 1/2, Enable Passthrough Case 0/2
  Enable Passthrough Case 0/1 -> Kernel Result Slice 1 Valid/1, Kernel Result Slice 0 Valid/1
  Enable Passthrough Case 1/1 -> Kernel Result Slice 3 Valid/1, Kernel Result Slice 2 Valid/1, Kernel Result Slice 4 Valid/1

== system CMOS_Kernel_Memory_Sync/Memory Handler/Math/Kernel Organizer/Determine Calculations Delay 1/Result Muxer 4 ==
  Select : Inport
  Valid : Inport  Port=2
  Case 0 : hdlBasic/Mux  inputs=2  en=off  latency=1  precision=Full  arith_type=Unsigned  n_bits=16  bin_pt=14  quantization=Truncate  overflow=Wrap  XmcBlockStatus=1  maskContainerNames=tabcontainer1  block_type=mux  block_config=sysgen:Mux_config
  Case 1 : hdlBasic/Mux  inputs=2  en=off  latency=1  precision=Full  arith_type=Unsigned  n_bits=16  bin_pt=14  quantization=Truncate  overflow=Wrap  XmcBlockStatus=1  maskContainerNames=tabcontainer1  block_type=mux  block_config=sysgen:Mux_config
  Delay Valid 0 : hdlBasic/Delay  rst=off  en=off  latency=1  reg_retiming=off  XmcBlockStatus=1  maskContainerNames=group1  block_type=delay  block_config=sysgen:Delay_config
  Enable Passthrough Case 0 : hdlBasic/Logical  logical_function=AND  inputs=2  en=off  latency=1  precision=Full  arith_type=Unsigned  n_bits=16  bin_pt=0  align_bp=on  overflow=[]  quantization=[]  XmcBlockStatus=1  maskContainerNames=tabcontainer1  block_type=logical  block_config=sysgen:Logical_config
  Enable Passthrough Case 1 : hdlBasic/Logical  logical_function=AND  inputs=2  en=off  latency=1  precision=Full  arith_type=Unsigned  n_bits=16  bin_pt=0  align_bp=on  overflow=[]  quantization=[]  XmcBlockStatus=1  maskContainerNames=tabcontainer1  block_type=logical  block_config=sysgen:Logical_config
  Off : hdlBasic/Constant  const=0  gui_display_data_type=Boolean  arith_type=Boolean  n_bits=16  bin_pt=14  preci_type=Single  exp_width=8  frac_width=24  explicit_period=off  period=1  XmcBlockStatus=1  maskContainerNames=tabcontainer1  block_type=constant  block_config=sysgen:Constant_config
  On : hdlBasic/Constant  const=1.0  gui_display_data_type=Boolean  arith_type=Boolean  n_bits=16  bin_pt=14  preci_type=Single  exp_width=8  frac_width=24  explicit_period=off  period=1  XmcBlockStatus=1  maskContainerNames=tabcontainer1  block_type=constant  block_config=sysgen:Constant_config
  Kernel Result Slice 0 Valid : Outport
  Kernel Result Slice 1 Valid : Outport  Port=2
  Kernel Result Slice 2 Valid : Outport  Port=3
  Kernel Result Slice 3 Valid : Outport  Port=4
  Kernel Result Slice 4 Valid : Outport  Port=5
  wires:
  Select/1 -> Case 0/1, Case 1/1
  On/1 -> Case 0/2, Case 1/3
  Off/1 -> Case 1/2, Case 0/3
  Valid/1 -> Delay Valid 0/1
  Case 0/1 -> Enable Passthrough Case 0/1
  Case 1/1 -> Enable Passthrough Case 1/1
  Delay Valid 0/1 -> Enable Passthrough Case 1/2, Enable Passthrough Case 0/2
  Enable Passthrough Case 0/1 -> Kernel Result Slice 0 Valid/1
  Enable Passthrough Case 1/1 -> Kernel Result Slice 4 Valid/1, Kernel Result Slice 1 Valid/1, Kernel Result Slice 2 Valid/1, Kernel Result Slice 3 Valid/1

== system CMOS_Kernel_Memory_Sync/Memory Handler/Math/Kernel Organizer/Determine Calculations Delay 1/Result Muxer 5 ==
  Select : Inport
  Valid : Inport  Port=2
  Force Off : Inport  Port=3
  Case 0 : hdlBasic/Mux  inputs=2  en=off  latency=1  precision=Full  arith_type=Unsigned  n_bits=16  bin_pt=14  quantization=Truncate  overflow=Wrap  XmcBlockStatus=1  maskContainerNames=tabcontainer1  block_type=mux  block_config=sysgen:Mux_config
  Case 1 : hdlBasic/Mux  inputs=2  en=off  latency=1  precision=Full  arith_type=Unsigned  n_bits=16  bin_pt=14  quantization=Truncate  overflow=Wrap  XmcBlockStatus=1  maskContainerNames=tabcontainer1  block_type=mux  block_config=sysgen:Mux_config
  Delay Valid 0 : hdlBasic/Delay  rst=off  en=off  latency=1  reg_retiming=off  XmcBlockStatus=1  maskContainerNames=group1  block_type=delay  block_config=sysgen:Delay_config
  Enable Passthrough Case 0 : hdlBasic/Logical  logical_function=AND  inputs=3  en=off  latency=1  precision=Full  arith_type=Unsigned  n_bits=16  bin_pt=0  align_bp=on  overflow=[]  quantization=[]  XmcBlockStatus=1  maskContainerNames=tabcontainer1  block_type=logical  block_config=sysgen:Logical_config
  Enable Passthrough Case 1 : hdlBasic/Logical  logical_function=AND  inputs=3  en=off  latency=1  precision=Full  arith_type=Unsigned  n_bits=16  bin_pt=0  align_bp=on  overflow=[]  quantization=[]  XmcBlockStatus=1  maskContainerNames=tabcontainer1  block_type=logical  block_config=sysgen:Logical_config
  Force Off MUX : hdlBasic/Mux  inputs=2  en=off  latency=1  precision=Full  arith_type=Unsigned  n_bits=16  bin_pt=14  quantization=Truncate  overflow=Wrap  XmcBlockStatus=1  maskContainerNames=tabcontainer1  block_type=mux  block_config=sysgen:Mux_config
  Off : hdlBasic/Constant  const=0  gui_display_data_type=Boolean  arith_type=Boolean  n_bits=16  bin_pt=14  preci_type=Single  exp_width=8  frac_width=24  explicit_period=off  period=1  XmcBlockStatus=1  maskContainerNames=tabcontainer1  block_type=constant  block_config=sysgen:Constant_config
  On : hdlBasic/Constant  const=1.0  gui_display_data_type=Boolean  arith_type=Boolean  n_bits=16  bin_pt=14  preci_type=Single  exp_width=8  frac_width=24  explicit_period=off  period=1  XmcBlockStatus=1  maskContainerNames=tabcontainer1  block_type=constant  block_config=sysgen:Constant_config
  Kernel Result Slice 0 Valid : Outport
  Kernel Result Slice 1 Valid : Outport  Port=2
  Kernel Result Slice 2 Valid : Outport  Port=3
  Kernel Result Slice 3 Valid : Outport  Port=4
  Kernel Result Slice 4 Valid : Outport  Port=5
  wires:
  Select/1 -> Case 0/1, Case 1/1
  Force Off/1 -> Force Off MUX/1
  On/1 -> Case 0/2, Force Off MUX/2, Case 1/3
  Off/1 -> Force Off MUX/3, Case 1/2, Case 0/3
  Valid/1 -> Delay Valid 0/1
  Case 0/1 -> Enable Passthrough Case 0/1
  Case 1/1 -> Enable Passthrough Case 1/1
  Delay Valid 0/1 -> Enable Passthrough Case 1/2, Enable Passthrough Case 0/2
  Force Off MUX/1 -> Enable Passthrough Case 0/3, Enable Passthrough Case 1/3
  Enable Passthrough Case 1/1 -> Kernel Result Slice 4 Valid/1, Kernel Result Slice 0 Valid/1, Kernel Result Slice 1 Valid/1, Kernel Result Slice 2 Valid/1, Kernel Result Slice 3 Valid/1

== system CMOS_Kernel_Memory_Sync/Memory Handler/Math/Kernel Organizer/Determine Calculations Delay 1/Result Muxer 6 ==
  Select : Inport
  Valid : Inport  Port=2
  Force Off : Inport  Port=3
  Force Off 2 : Inport  Port=4
  Case 0 : hdlBasic/Mux  inputs=2  en=off  latency=1  precision=Full  arith_type=Unsigned  n_bits=16  bin_pt=14  quantization=Truncate  overflow=Wrap  XmcBlockStatus=1  maskContainerNames=tabcontainer1  block_type=mux  block_config=sysgen:Mux_config
  Case 1 : hdlBasic/Mux  inputs=2  en=off  latency=1  precision=Full  arith_type=Unsigned  n_bits=16  bin_pt=14  quantization=Truncate  overflow=Wrap  XmcBlockStatus=1  maskContainerNames=tabcontainer1  block_type=mux  block_config=sysgen:Mux_config
  Delay Valid 0 : hdlBasic/Delay  rst=off  en=off  latency=1  reg_retiming=off  XmcBlockStatus=1  maskContainerNames=group1  block_type=delay  block_config=sysgen:Delay_config
  Enable Passthrough Case 0 : hdlBasic/Logical  logical_function=AND  inputs=4  en=off  latency=1  precision=Full  arith_type=Unsigned  n_bits=16  bin_pt=0  align_bp=on  overflow=[]  quantization=[]  XmcBlockStatus=1  maskContainerNames=tabcontainer1  block_type=logical  block_config=sysgen:Logical_config
  Enable Passthrough Case 1 : hdlBasic/Logical  logical_function=AND  inputs=4  en=off  latency=1  precision=Full  arith_type=Unsigned  n_bits=16  bin_pt=0  align_bp=on  overflow=[]  quantization=[]  XmcBlockStatus=1  maskContainerNames=tabcontainer1  block_type=logical  block_config=sysgen:Logical_config
  Force Off MUX : hdlBasic/Mux  inputs=2  en=off  latency=1  precision=Full  arith_type=Unsigned  n_bits=16  bin_pt=14  quantization=Truncate  overflow=Wrap  XmcBlockStatus=1  maskContainerNames=tabcontainer1  block_type=mux  block_config=sysgen:Mux_config
  Force Off MUX1 : hdlBasic/Mux  inputs=2  en=off  latency=1  precision=Full  arith_type=Unsigned  n_bits=16  bin_pt=14  quantization=Truncate  overflow=Wrap  XmcBlockStatus=1  maskContainerNames=tabcontainer1  block_type=mux  block_config=sysgen:Mux_config
  Off : hdlBasic/Constant  const=0  gui_display_data_type=Boolean  arith_type=Boolean  n_bits=16  bin_pt=14  preci_type=Single  exp_width=8  frac_width=24  explicit_period=off  period=1  XmcBlockStatus=1  maskContainerNames=tabcontainer1  block_type=constant  block_config=sysgen:Constant_config
  On : hdlBasic/Constant  const=1.0  gui_display_data_type=Boolean  arith_type=Boolean  n_bits=16  bin_pt=14  preci_type=Single  exp_width=8  frac_width=24  explicit_period=off  period=1  XmcBlockStatus=1  maskContainerNames=tabcontainer1  block_type=constant  block_config=sysgen:Constant_config
  Kernel Result Slice 0 Valid : Outport
  Kernel Result Slice 1 Valid : Outport  Port=2
  Kernel Result Slice 2 Valid : Outport  Port=3
  Kernel Result Slice 3 Valid : Outport  Port=4
  Kernel Result Slice 4 Valid : Outport  Port=5
  wires:
  Select/1 -> Case 0/1, Case 1/1
  Force Off/1 -> Force Off MUX/1
  On/1 -> Case 0/2, Force Off MUX/2, Force Off MUX1/2, Case 1/3
  Off/1 -> Force Off MUX1/3, Force Off MUX/3, Case 1/2, Case 0/3
  Valid/1 -> Delay Valid 0/1
  Case 0/1 -> Enable Passthrough Case 0/1
  Case 1/1 -> Enable Passthrough Case 1/1
  Delay Valid 0/1 -> Enable Passthrough Case 1/2, Enable Passthrough Case 0/2
  Force Off MUX/1 -> Enable Passthrough Case 0/3, Enable Passthrough Case 1/3
  Enable Passthrough Case 1/1 -> Kernel Result Slice 0 Valid/1, Kernel Result Slice 1 Valid/1, Kernel Result Slice 2 Valid/1, Kernel Result Slice 3 Valid/1
  Enable Passthrough Case 0/1 -> Kernel Result Slice 4 Valid/1
  Force Off 2/1 -> Force Off MUX1/1
  Force Off MUX1/1 -> Enable Passthrough Case 1/4, Enable Passthrough Case 0/4

== system CMOS_Kernel_Memory_Sync/Memory Handler/Math/Kernel Organizer/Determine Calculations Delay 1/Result Muxer 7 ==
  Select : Inport
  Valid : Inport  Port=2
  Force Off : Inport  Port=3
  Force Off 2 : Inport  Port=4
  Case 0 : hdlBasic/Mux  inputs=2  en=off  latency=1  precision=Full  arith_type=Unsigned  n_bits=16  bin_pt=14  quantization=Truncate  overflow=Wrap  XmcBlockStatus=1  maskContainerNames=tabcontainer1  block_type=mux  block_config=sysgen:Mux_config
  Case 1 : hdlBasic/Mux  inputs=2  en=off  latency=1  precision=Full  arith_type=Unsigned  n_bits=16  bin_pt=14  quantization=Truncate  overflow=Wrap  XmcBlockStatus=1  maskContainerNames=tabcontainer1  block_type=mux  block_config=sysgen:Mux_config
  Delay Valid 0 : hdlBasic/Delay  rst=off  en=off  latency=1  reg_retiming=off  XmcBlockStatus=1  maskContainerNames=group1  block_type=delay  block_config=sysgen:Delay_config
  Enable Passthrough Case 0 : hdlBasic/Logical  logical_function=AND  inputs=4  en=off  latency=1  precision=Full  arith_type=Unsigned  n_bits=16  bin_pt=0  align_bp=on  overflow=[]  quantization=[]  XmcBlockStatus=1  maskContainerNames=tabcontainer1  block_type=logical  block_config=sysgen:Logical_config
  Enable Passthrough Case 1 : hdlBasic/Logical  logical_function=AND  inputs=4  en=off  latency=1  precision=Full  arith_type=Unsigned  n_bits=16  bin_pt=0  align_bp=on  overflow=[]  quantization=[]  XmcBlockStatus=1  maskContainerNames=tabcontainer1  block_type=logical  block_config=sysgen:Logical_config
  Force Off MUX : hdlBasic/Mux  inputs=2  en=off  latency=1  precision=Full  arith_type=Unsigned  n_bits=16  bin_pt=14  quantization=Truncate  overflow=Wrap  XmcBlockStatus=1  maskContainerNames=tabcontainer1  block_type=mux  block_config=sysgen:Mux_config
  Force Off MUX1 : hdlBasic/Mux  inputs=2  en=off  latency=1  precision=Full  arith_type=Unsigned  n_bits=16  bin_pt=14  quantization=Truncate  overflow=Wrap  XmcBlockStatus=1  maskContainerNames=tabcontainer1  block_type=mux  block_config=sysgen:Mux_config
  Off : hdlBasic/Constant  const=0  gui_display_data_type=Boolean  arith_type=Boolean  n_bits=16  bin_pt=14  preci_type=Single  exp_width=8  frac_width=24  explicit_period=off  period=1  XmcBlockStatus=1  maskContainerNames=tabcontainer1  block_type=constant  block_config=sysgen:Constant_config
  On : hdlBasic/Constant  const=1.0  gui_display_data_type=Boolean  arith_type=Boolean  n_bits=16  bin_pt=14  preci_type=Single  exp_width=8  frac_width=24  explicit_period=off  period=1  XmcBlockStatus=1  maskContainerNames=tabcontainer1  block_type=constant  block_config=sysgen:Constant_config
  Kernel Result Slice 0 Valid : Outport
  Kernel Result Slice 1 Valid : Outport  Port=2
  Kernel Result Slice 2 Valid : Outport  Port=3
  Kernel Result Slice 3 Valid : Outport  Port=4
  Kernel Result Slice 4 Valid : Outport  Port=5
  wires:
  Select/1 -> Case 0/1, Case 1/1
  Force Off/1 -> Force Off MUX/1
  On/1 -> Case 0/2, Force Off MUX/2, Force Off MUX1/2, Case 1/3
  Off/1 -> Force Off MUX1/3, Force Off MUX/3, Case 1/2, Case 0/3
  Valid/1 -> Delay Valid 0/1
  Case 0/1 -> Enable Passthrough Case 0/1
  Case 1/1 -> Enable Passthrough Case 1/1
  Delay Valid 0/1 -> Enable Passthrough Case 1/2, Enable Passthrough Case 0/2
  Force Off MUX/1 -> Enable Passthrough Case 0/3, Enable Passthrough Case 1/3
  Enable Passthrough Case 1/1 -> Kernel Result Slice 0 Valid/1, Kernel Result Slice 1 Valid/1, Kernel Result Slice 2 Valid/1
  Enable Passthrough Case 0/1 -> Kernel Result Slice 3 Valid/1, Kernel Result Slice 4 Valid/1
  Force Off 2/1 -> Force Off MUX1/1
  Force Off MUX1/1 -> Enable Passthrough Case 0/4, Enable Passthrough Case 1/4
